simulink model "M182_Lab4"  (R2019b)
settings: Solver=VariableStepAuto  StartTime=0.0  StopTime=30  RelTol=1e-3
settings Model: Creator=scjcb  LastModifiedBy=scjcb

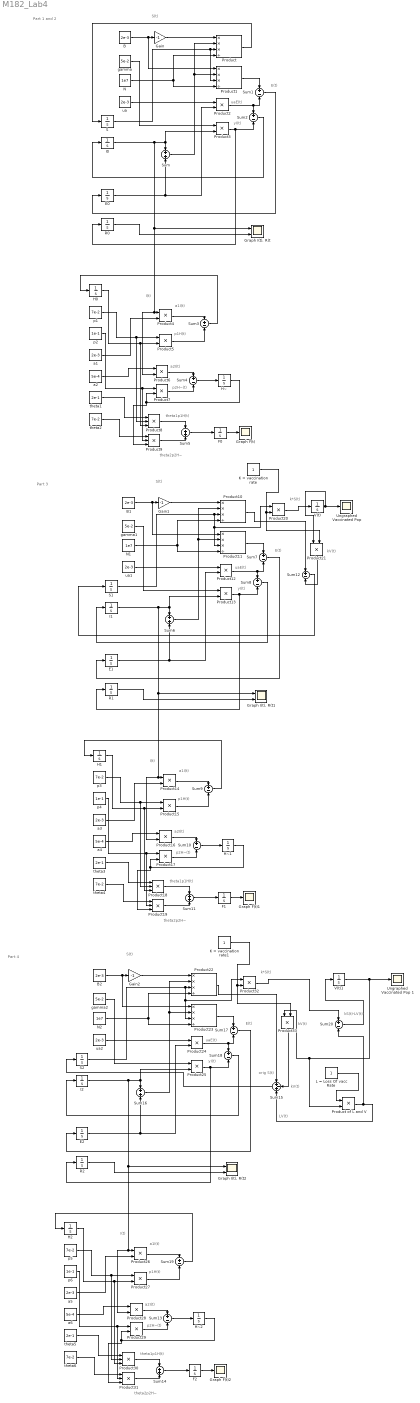
== system M182_Lab4 ==
  note: LV(t)
  note: kV(t)
  note: orig S(t)
  note: kS(t)-LV(t)
  note: kV(t)
  note: k*S(t)
  note: Part 1 and 2
  note: I(t)
  note: p2H~(t)
  note: a2I(t)
  note: theta2p2H~
  note: theta1p1H(t)
  note: p1H(t)
  note: a1I(t)
  note: uaE(t)
  note: yI(t)
  note: E(t)
  note: S(t)
  note: Part 3
  note: p2H~(t)
  note: theta2p2H~
  note: I(t)
  note: uaE(t)
  note: p1H(t)
  note: theta1p1H(t)
  note: a2I(t)
  note: yI(t)
  note: E(t)
  note: a1I(t)
  note: S(t)
  note: kV(t)
  note: S(t)
  note: theta1p1H(t)
  note: yI(t)
  note: Part 4
  note: p2H~(t)
  note: I(t)
  note: a2I(t)
  note: theta2p2H~
  note: E(t)
  note: uaE(t)
  note: k*S(t)
  note: a1I(t)
  note: p1H(t)
  B : Constant  Value=2e-3
  B1 : Constant  Value=2e-3
  B2 : Constant  Value=2e-3
  E0 : Integrator  InitialCondition=6e5
  E1 : Integrator  InitialCondition=6e5
  E2 : Integrator  InitialCondition=6e5
  F0 : Integrator  InitialCondition=6.5e3
  F1 : Integrator  InitialCondition=6.5e3
  F2 : Integrator  InitialCondition=6.5e3
  Gain : Gain  Gain=-1
  Gain1 : Gain  Gain=-1
  Gain2 : Gain  Gain=-1
  Graph F(t) : Scope
  Graph F(t)1 : Scope
  Graph F(t)2 : Scope
  "Graph I(t), R(t" : Scope  NumInputPorts=2
  "Graph I(t), R(t1" : Scope  NumInputPorts=2
  "Graph I(t), R(t2" : Scope  NumInputPorts=2
  H0 : Integrator  InitialCondition=7e2
  H1 : Integrator  InitialCondition=7e2
  H2 : Integrator  InitialCondition=7e2
  H~ : Integrator  InitialCondition=188
  H~1 : Integrator  InitialCondition=188
  H~2 : Integrator  InitialCondition=188
  I0 : Integrator  InitialCondition=3e4
  I1 : Integrator  InitialCondition=3e4
  I2 : Integrator  InitialCondition=3e4
  K = vaccination rate : Constant
  K = vaccination rate1 : Constant
  L = Loss Of vacc Rate : Constant
  N : Constant  Value=1e7
  N1 : Constant  Value=1e7
  N2 : Constant  Value=1e7
  Product{,1,10..11,22..23} (6 alike) : Product  Inputs=***/
  Product of L and V : Product  Inputs=**
  Product{2,4..7,12,14..17,20..21,24,26..29,32..33} (19 alike) : Product  Inputs=**
  Product13 : Product
  Product{8..9,18..19,30..31} (6 alike) : Product  Inputs=***
  Product25 : Product
  Product3 : Product
  R0 : Integrator  InitialCondition=2.3e5
  R1 : Integrator  InitialCondition=2.3e5
  R2 : Integrator  InitialCondition=2.3e5
  S : Integrator  InitialCondition=9e6
  S1 : Integrator  InitialCondition=9e6
  S2 : Integrator  InitialCondition=9e6
  Sum{,5..6,11,14,16} (6 alike) : Sum
  Sum{1..4,7..10,12..13,17..20} (14 alike) : Sum  Inputs=+-
  Sum15 : Sum  Inputs=+-+
  "Ungraphed Vaccinated Pop " : Scope
  Ungraphed Vaccinated Pop 1 : Scope
  V(t) : Integrator
  V(t)1 : Integrator
  a1 : Constant  Value=2e-3
  a2 : Constant  Value=5e-4
  a3 : Constant  Value=2e-3
  a4 : Constant  Value=5e-4
  a5 : Constant  Value=2e-3
  a6 : Constant  Value=5e-4
  gamma : Constant  Value=5e-2
  gamma1 : Constant  Value=5e-2
  gamma2 : Constant  Value=5e-2
  p1 : Constant  Value=7e-2
  p2 : Constant  Value=1e-1
  p3 : Constant  Value=7e-2
  p4 : Constant  Value=1e-1
  p5 : Constant  Value=7e-2
  p6 : Constant  Value=1e-1
  theta1 : Constant  Value=2e-1
  theta2 : Constant  Value=7e-2
  theta3 : Constant  Value=2e-1
  theta4 : Constant  Value=7e-2
  theta5 : Constant  Value=2e-1
  theta6 : Constant  Value=7e-2
  ua : Constant  Value=2e-3
  ua1 : Constant  Value=2e-3
  ua2 : Constant  Value=2e-3
  wires:
  N/1 -> Product1/4, Product/4
  B/1 -> Product1/1, Gain/1
  I0/1 -> "Graph I(t), R(t"/1, Product6/2, Product4/1, Product3/2, Sum/1
  E0/1 -> Sum/2, Product2/2
  Gain/1 -> Product/1
  Sum/1 -> Product1/2, Product/2
  S/1 -> Product1/3, Product/3
  Product/1 -> S/1
  ua/1 -> Product2/1
  Product1/1 -> Sum1/1
  Product2/1 -> Sum2/1, Sum1/2
  Sum1/1 -> E0/1
  gamma/1 -> Product3/1
  Product3/1 -> R0/1, Sum2/2
  Sum2/1 -> I0/1
  a1/1 -> Product4/2
  p1/1 -> Product5/1, Product8/2
  H0/1 -> Product5/2, Product8/3
  Product4/1 -> Sum3/1
  Product5/1 -> Sum3/2
  Sum3/1 -> H0/1
  a2/1 -> Product6/1
  Product6/1 -> Sum4/1
  Product7/1 -> Sum4/2
  Sum4/1 -> H~/1
  H~/1 -> Product9/3, Product7/2
  theta1/1 -> Product8/1
  theta2/1 -> Product9/1
  p2/1 -> Product9/2, Product7/1
  Product8/1 -> Sum5/1
  Product9/1 -> Sum5/2
  Sum5/1 -> F0/1
  F0/1 -> Graph F(t)/1
  R0/1 -> "Graph I(t), R(t"/2
  a3/1 -> Product14/2
  Product13/1 -> R1/1, Sum8/2
  p4/1 -> Product19/2, Product17/1
  S1/1 -> Product11/3, Product20/1, Product10/3
  Product10/1 -> Sum12/1
  ua1/1 -> Product12/1
  E1/1 -> Sum6/2, Product12/2
  I1/1 -> "Graph I(t), R(t1"/1, Product16/2, Product14/1, Product13/2, Sum6/1
  theta3/1 -> Product18/1
  Product14/1 -> Sum9/1
  B1/1 -> Product11/1, Gain1/1
  Product19/1 -> Sum11/2
  Sum6/1 -> Product11/2, Product10/2
  R1/1 -> "Graph I(t), R(t1"/2
  Gain1/1 -> Product10/1
  Sum10/1 -> H~1/1
  Sum8/1 -> I1/1
  H~1/1 -> Product19/3, Product17/2
  Product17/1 -> Sum10/2
  N1/1 -> Product11/4, Product10/4
  p3/1 -> Product15/1, Product18/2
  Product18/1 -> Sum11/1
  Sum11/1 -> F1/1
  H1/1 -> Product15/2, Product18/3
  Product11/1 -> Sum7/1
  F1/1 -> Graph F(t)1/1
  theta4/1 -> Product19/1
  Product12/1 -> Sum8/1, Sum7/2
  Product15/1 -> Sum9/2
  gamma1/1 -> Product13/1
  Sum7/1 -> E1/1
  a4/1 -> Product16/1
  Sum9/1 -> H1/1
  Product16/1 -> Sum10/1
  K = vaccination rate/1 -> Product21/2, Product20/2
  Product20/1 -> V(t)/1
  V(t)/1 -> Product21/1, "Ungraphed Vaccinated Pop "/1
  Product21/1 -> Sum12/2
  Sum12/1 -> S1/1
  Product32/1 -> Sum20/1
  K = vaccination rate1/1 -> Product33/2, Product32/2
  Product28/1 -> Sum13/1
  Sum17/1 -> E2/1
  Sum19/1 -> H2/1
  a6/1 -> Product28/1
  Product23/1 -> Sum17/1
  F2/1 -> Graph F(t)2/1
  H2/1 -> Product27/2, Product30/3
  Sum14/1 -> F2/1
  R2/1 -> "Graph I(t), R(t2"/2
  Product31/1 -> Sum14/2
  V(t)1/1 -> Ungraphed Vaccinated Pop 1/1, Product of L and V/2, Product33/1
  Sum15/1 -> S2/1
  B2/1 -> Product23/1, Gain2/1
  I2/1 -> "Graph I(t), R(t2"/1, Product28/2, Product26/1, Product25/2, Sum16/1
  Product26/1 -> Sum19/1
  theta5/1 -> Product30/1
  Sum16/1 -> Product23/2, Product22/2
  Product27/1 -> Sum19/2
  Product22/1 -> Sum15/1
  S2/1 -> Product23/3, Product32/1, Product22/3
  E2/1 -> Sum16/2, Product24/2
  p6/1 -> Product31/2, Product29/1
  ua2/1 -> Product24/1
  theta6/1 -> Product31/1
  Product25/1 -> R2/1, Sum18/2
  a5/1 -> Product26/2
  Product33/1 -> Sum15/2
  gamma2/1 -> Product25/1
  p5/1 -> Product27/1, Product30/2
  Product30/1 -> Sum14/1
  N2/1 -> Product23/4, Product22/4
  H~2/1 -> Product31/3, Product29/2
  Gain2/1 -> Product22/1
  Product29/1 -> Sum13/2
  Sum13/1 -> H~2/1
  Product24/1 -> Sum18/1, Sum17/2
  Sum18/1 -> I2/1
  L = Loss Of vacc Rate/1 -> Product of L and V/1
  Product of L and V/1 -> Sum15/3, Sum20/2
  Sum20/1 -> V(t)1/1
